simulink library "vmc"  (R2021b)
settings: Solver=VariableStepAuto  StartTime=0.0  StopTime=10.0  RelTol=1e-3
undefined symbols (not defined in the file or in its folder): AVMC_ACCDeltaTqIGain4OVRD_X_kph, AVMC_ACCDeltaTqIGain4OVRD_Y_mps2, AVMC_ACCDeltaTqIGain_X_kph, AVMC_ACCDeltaTqIGain_Y_mps2, AVMC_ACCDeltaTqPGain_X_kph, AVMC_ACCDeltaTqPGain_Y_kph, AVMC_ACCLongSteadyCtrl_X_kph, AVMC_ADSPosGFBDeltaTq_X_kph, AVMC_ADSPosGFBDeltaTq_Y_mps2, AVMC_AggressJerkPCT4AT_X_kph, AVMC_AggressJerkPCT_X_kph, AVMC_AggressLimitPCT4AT_X_kph, AVMC_AggressLimitPCT_X_kph, AVMC_CCLongSteadyCtrl_X_kph, AVMC_DISCDeltaTqIGain_X_kph, AVMC_DISCDeltaTqIGain_Y_mps2, AVMC_DISCDeltaTqPGain_X_kph, AVMC_DISCDeltaTqPGain_Y_kph, AVMC_ESCRegenOut_X_kph, AVMC_ESCRegenOut_Y_Deg, AVMC_ESCRegenOutEnSpd_X_Deg, AVMC_ISOAccLimit_X_mps, AVMC_ISODecLimit_X_mps, AVMC_ISOJerk_X_mps, AVMC_LatESCRegenOut_X_kph, AVMC_LatESCRegenOut_Y_Deg, AVMC_LongAccDeadZone_X_kph, AVMC_LongAccFiltTsforP2_X_Gps, AVMC_MCPresBaseTq_X_bar, AVMC_MSALongSteadyCtrl_X_kph, AVMC_MSAPedalOvrd_X_kph, AVMC_MSASpdBand_X_kph, AVMC_MSATqDownEndTq_X_kph, AVMC_MSATqDownTime_X_kph, AVMC_OPDDisSlideRate_X_Deg, AVMC_OVRD2ActSR2FCMCMD_X_mps2, AVMC_PedalTqRWhlRatio_X_Nm, AVMC_PedalTqRWhlRatio_Y_gps, AVMC_PedalTqRWhlSlipGain_X_rat, AVMC_PedalTqRWhlSlipGain_Y_kph, AVMC_PedalTqRWhSTRGGain_X_deg, AVMC_PedalTqRWhSTRGGain_Y_kph, AVMC_RDCDetectTime_X_kph, AVMC_RDCDetectTime_Y_pct, AVMC_RDCEnSlideRate_X_Deg, AVMC_RearWhlTqRatio_X_Nm, AVMC_RearWhlTqRatio_Y_gps, AVMC_RearWhlTqSlipGain_X_rat, AVMC_RearWhlTqSlipGain_Y_kph, AVMC_RearWhlTqSTRGGain_X_deg, AVMC_RearWhlTqSTRGGain_Y_kph, AVMC_ReqBrkJoinDecSR_X_mps2, AVMC_SoftJerkPCT_X_kph, AVMC_SoftLimitPCT_X_kph, AVMC_StESCYaw_X_kph, AVMC_StESCYaw_Y_Deg, AVMC_StESCYawCom_X_kph, AVMC_StESCYawCom_Y_Gps, AVMC_TMSpdBaseTq_X_rpm, AVMC_VehHoldDecCtrlTime2_X_kph ... (+411)
libraries: hcu_lib x108, simulink x82, tqr x1, simulink_extras x1
(part 3 of 14)

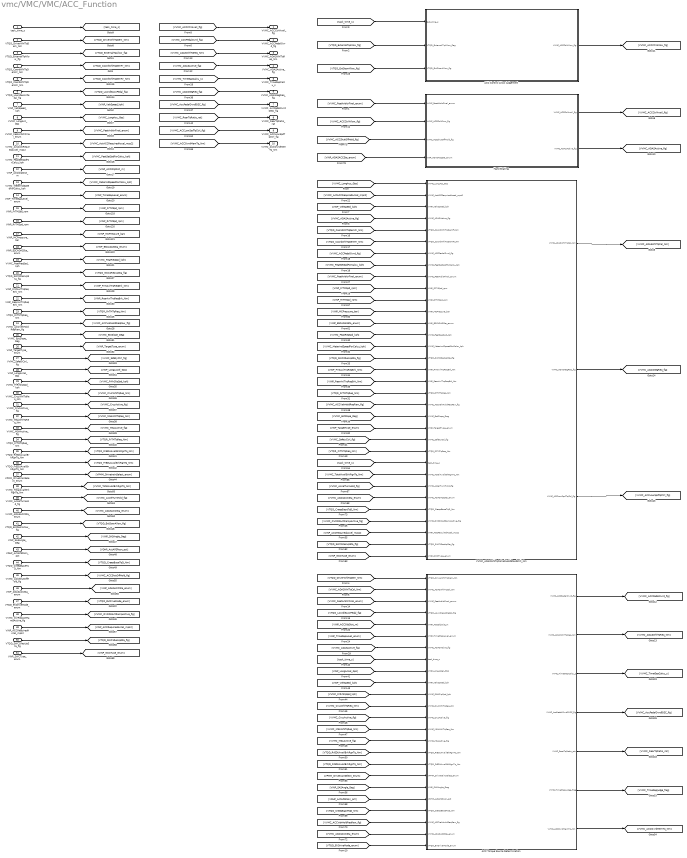
== system vmc/VMC/VMC/ACC_Function ==
  task_time_s : Inport
  VTQD_DriverWhlTqDem_Nm : Inport  Port=2
  VTQD_ExternalTqAllow_flg : Inport  Port=3
  VTQD_CoordWhlTqDemFr_Nm : Inport  Port=4
  VTQD_CoordWhlTqDemRr_Nm : Inport  Port=5
  VTQD_LowIdleAccPedal_flg : Inport  Port=6
  VINP_VehSpeed_kph : Inport  Port=7
  VVMC_LongAcc_Gps : Inport  Port=8
  VVMC_FeatArbitrFinal_enum : Inport  Port=9
  VVMC_ActACCRequiredAccel_mps2 : Inport  Port=10
  VVMC_FeatSetSpdForCalcu_kph : Inport  Port=11
  VINP_ACCObjDist_m : Inport  Port=12
  VVMC_MeterIndSpeedForCalcu_kph : Inport  Port=13
  VINP_TimeGapLevel_enum : Inport  Port=14
  VINP_FrTMSpd_rpm : Inport  Port=15
  VINP_RrTMSpd_rpm : Inport  Port=16
  VINP_MCPressure_bar : Inport  Port=17
  VINP_ESCADASSta_enum : Inport  Port=18
  VVMC_FeatReqSpd_kph : Inport  Port=19
  VTQD_SWC2ResUpSta_flg : Inport  Port=20
  VINP_FrntAxlTrqReqBrk_Nm : Inport  Port=21
  VINP_RearAxlTrqReqBrk_Nm : Inport  Port=22
  VTQR_RrTMTqReq_Nm : Inport  Port=23
  VVMC_ACCVehHoldReqRaw_flg : Inport  Port=24
  VVMC_EstSlope_Deg : Inport  Port=25
  VINP_TargetType_enum : Inport  Port=26
  VVMC_SafetyCtrl_flg : Inport  Port=27
  VINP_LongAccel_Gps : Inport  Port=28
  VVMC_FrRrSlipSpd_kph : Inport  Port=29
  VVMC_CruzWhlTqReq_Nm : Inport  Port=30
  VVMC_CruzActive_flg : Inport  Port=31
  VVMC_MSAWhlTqReq_Nm : Inport  Port=32
  VVMC_MSAActive_flg : Inport  Port=33
  VTQR_FrTMTqReq_Nm : Inport  Port=34
  VTQD_RrEDUAvailBrkRgnTq_Nm : Inport  Port=35
  VTQD_FrEDUAvailBrkRgnTq_Nm : Inport  Port=36
  VPMM_DrivetrainSelect_enum : Inport  Port=37
  VVMC_TotalAvailBrkRgnTq_Nm : Inport  Port=38
  VVMC_AccelTurnHold_flg : Inport  Port=39
  VVMC_ADASACCSta_enum : Inport  Port=40
  VTQD_ExtDoorAllow_flg : Inport  Port=41
  VINP_SASAngle_Deg : Inport  Port=42
  VDHP_ActAPSPosn_pct : Inport  Port=43
  VTQD_CreepBaseTqD_Nm : Inport  Port=44
  VVMC_ACCShutOffHold_flg : Inport  Port=45
  VINP_ADASACCSta_enum : Inport  Port=46
  VTQD_EVDriveMode_enum : Inport  Port=47
  VVMC_OVRD2ActRampActive_flg : Inport  Port=48
  VINP_ACCRequiredAccel_mps2 : Inport  Port=49
  VTQD_SWC1ResUpSta_flg : Inport  Port=50
  VINP_SWCType_enum : Inport  Port=51
  ACC Control Allow Judgement : Subsystem
  ACC Torque Source Determination : Subsystem
  Hand Shaking : Subsystem
  VVMC_ADASWhlTqCalVehHoldStandstill_Nm : Subsystem
  VVMC_ACCCtrlAvail_flg : Outport
  VVMC_ACCPedalOvrd_flg : Outport  Port=2
  VVMC_ADASWhlTqReq_Nm : Outport  Port=3
  VVMC_ADASActive_flg : Outport  Port=4
  VVMC_TimeGapCalcu_s : Outport  Port=5
  VVMC_ADASNegReq_flg : Outport  Port=6
  VVMC_AccPedalOvrdDISC_flg : Outport  Port=7
  VVMC_RearTqRatio_rat : Outport  Port=8
  VVMC_ACCLowSpdTqCtrl_flg : Outport  Port=9
  VVMC_ACCOvrdMemTq_Nm : Outport  Port=10
  wires:
  [VVMC_FeatReqSpd_kph] -> VVMC_ADASWhlTqCalVehHoldStandstill_Nm/14(VVMC_FeatReqSpd_kph)
  VVMC_FeatReqSpd_kph/1 -> [VVMC_FeatReqSpd_kph]
  [VVMC_ADASActive_flg] -> ACC Torque Source Determination/7(VVMC_ADASActive_flg)
  [VINP_ESCADASSta_enum] -> VVMC_ADASWhlTqCalVehHoldStandstill_Nm/13(VINP_ESCADASSta_enum)
  [VINP_MCPressure_bar] -> VVMC_ADASWhlTqCalVehHoldStandstill_Nm/12(VINP_MCPressure_bar)
  [VINP_RrTMSpd_rpm] -> VVMC_ADASWhlTqCalVehHoldStandstill_Nm/11(VINP_RrTMSpd_rpm)
  [VINP_FrTMSpd_rpm] -> VVMC_ADASWhlTqCalVehHoldStandstill_Nm/10(VINP_FrTMSpd_rpm)
  VINP_FrTMSpd_rpm/1 -> [VINP_FrTMSpd_rpm]
  VINP_RrTMSpd_rpm/1 -> [VINP_RrTMSpd_rpm]
  VINP_MCPressure_bar/1 -> [VINP_MCPressure_bar]
  VINP_ESCADASSta_enum/1 -> [VINP_ESCADASSta_enum]
  [VVMC_FeatArbitrFinal_enum] -> VVMC_ADASWhlTqCalVehHoldStandstill_Nm/9(VVMC_FeatArbitrFinal_enum)
  [VTQD_ExternalTqAllow_flg] -> ACC Control Allow Judgement/2(VTQD_ExternalTqAllow_flag)
  ACC Control Allow Judgement/1(VVMC_ACCCtrlAllow_flg) -> [VVMC_ACCCtrlAllow_flg]
  [task_time_s] -> ACC Control Allow Judgement/1(task_time_s)
  [VVMC_TimeGapCalcu_s] -> VVMC_TimeGapCalcu_s/1
  ACC Torque Source Determination/3(VVMC_TimeGapCalcu_s) -> [VVMC_TimeGapCalcu_s]
  [VINP_TimeGapLevel_enum] -> ACC Torque Source Determination/6(VINP_TimeGapLevel_enum)
  [VINP_ACCObjDist_m] -> ACC Torque Source Determination/5(VINP_ACCObjDist_m)
  VINP_TimeGapLevel_enum/1 -> [VINP_TimeGapLevel_enum]
  VINP_ACCObjDist_m/1 -> [VINP_ACCObjDist_m]
  VVMC_MeterIndSpeedForCalcu_kph/1 -> [VVMC_MeterIndSpeedForCalcu_kph]
  [VVMC_ACCPedalOvrd_flg] -> VVMC_ACCPedalOvrd_flg/1
  Hand Shaking/1(VVMC_ACCCtrlAvail_flg) -> [VVMC_ACCCtrlAvail_flg]
  VVMC_LongAcc_Gps/1 -> [VVMC_LongAcc_Gps]
  VVMC_FeatArbitrFinal_enum/1 -> [VVMC_FeatArbitrFinal_enum]
  VVMC_ActACCRequiredAccel_mps2/1 -> [VVMC_ActACCRequiredAccel_mps2]
  [VVMC_ACCCtrlAvail_flg] -> VVMC_ACCCtrlAvail_flg/1
  VTQD_ExternalTqAllow_flg/1 -> [VTQD_ExternalTqAllow_flg]
  VINP_VehSpeed_kph/1 -> [VINP_VehSpeed_kph]
  VTQD_DriverWhlTqDem_Nm/1 -> [VTQD_DriverWhlTqDem_Nm]
  [VVMC_LongAcc_Gps] -> VVMC_ADASWhlTqCalVehHoldStandstill_Nm/1(VVMC_LongAcc_Gps)
  [VVMC_ActACCRequiredAccel_mps2] -> VVMC_ADASWhlTqCalVehHoldStandstill_Nm/2(VVMC_ActACCRequiredAccel_mps2)
  [VINP_VehSpeed_kph] -> VVMC_ADASWhlTqCalVehHoldStandstill_Nm/3(VINP_VehSpeed_kph)
  VVMC_ADASWhlTqCalVehHoldStandstill_Nm/1(VVMC_ADASWhlTqCal_Nm) -> [VVMC_ADASWhlTqCal_Nm]
  [VTQD_DriverWhlTqDem_Nm] -> ACC Torque Source Determination/1(VTQD_DriverWhlTqDem_Nm)
  [VVMC_ADASWhlTqCal_Nm] -> ACC Torque Source Determination/2(VVMC_ADASWhlTqCal_Nm)
  ACC Torque Source Determination/1(VVMC_ACCPedalOvrd_flg) -> [VVMC_ACCPedalOvrd_flg]
  [VVMC_FeatArbitrFinal_enum] -> Hand Shaking/1(VVMC_FeatArbitrFinal_enum)
  Hand Shaking/2(VVMC_ADASActive_flg) -> [VVMC_ADASActive_flg]
  [VVMC_ADASActive_flg] -> VVMC_ADASWhlTqCalVehHoldStandstill_Nm/4(VVMC_ADASActive_flg)
  task_time_s/1 -> [task_time_s]
  [VVMC_ACCCtrlAllow_flg] -> Hand Shaking/2(VVMC_ACCCtrlAllow_flg)
  [VVMC_ADASActive_flg] -> VVMC_ADASActive_flg/1
  ACC Torque Source Determination/2(VVMC_ADASWhlTqReq_Nm) -> [VVMC_ADASWhlTqReq_Nm]
  [VVMC_ADASWhlTqReq_Nm] -> VVMC_ADASWhlTqReq_Nm/1
  [VTQD_CoordWhlTqDemFr_Nm] -> VVMC_ADASWhlTqCalVehHoldStandstill_Nm/5(VTQD_CoordWhlTqDemFr_Nm)
  [VTQD_CoordWhlTqDemRr_Nm] -> VVMC_ADASWhlTqCalVehHoldStandstill_Nm/6(VTQD_CoordWhlTqDemRr_Nm)
  VTQD_CoordWhlTqDemRr_Nm/1 -> [VTQD_CoordWhlTqDemRr_Nm]
  VTQD_CoordWhlTqDemFr_Nm/1 -> [VTQD_CoordWhlTqDemFr_Nm]
  [VVMC_ACCPedalOvrd_flg] -> VVMC_ADASWhlTqCalVehHoldStandstill_Nm/7(VVMC_ACCPedalOvrd_flg)
  [VVMC_FeatArbitrFinal_enum] -> ACC Torque Source Determination/3(VVMC_FeatArbitrFinal_enum)
  VTQD_LowIdleAccPedal_flg/1 -> [VTQD_LowIdleAccPedal_flg]
  [VTQD_LowIdleAccPedal_flg] -> ACC Torque Source Determination/4(VTQD_LowIdleAccPedal_flg)
  VVMC_FeatSetSpdForCalcu_kph/1 -> [VVMC_FeatSetSpdForCalcu_kph]
  [VVMC_FeatSetSpdForCalcu_kph] -> VVMC_ADASWhlTqCalVehHoldStandstill_Nm/8(VVMC_FeatSetSpdForCalcu_kph)
  VTQD_SWC2ResUpSta_flg/1 -> [VTQD_SWC2ResUpSta_flg]
  VINP_FrntAxlTrqReqBrk_Nm/1 -> [VINP_FrntAxlTrqReqBrk_Nm]
  VINP_RearAxlTrqReqBrk_Nm/1 -> [VINP_RearAxlTrqReqBrk_Nm]
  [VVMC_MeterIndSpeedForCalcu_kph] -> VVMC_ADASWhlTqCalVehHoldStandstill_Nm/15(VVMC_MeterIndSpeedForCalcu_kph)
  [VTQD_SWC2ResUpSta_flg] -> VVMC_ADASWhlTqCalVehHoldStandstill_Nm/16(VTQD_SWC2ResUpSta_flg)
  [VINP_FrntAxlTrqReqBrk_Nm] -> VVMC_ADASWhlTqCalVehHoldStandstill_Nm/17(VINP_FrntAxlTrqReqBrk_Nm)
  [VINP_RearAxlTrqReqBrk_Nm] -> VVMC_ADASWhlTqCalVehHoldStandstill_Nm/18(VINP_RearAxlTrqReqBrk_Nm)
  VVMC_ADASWhlTqCalVehHoldStandstill_Nm/2(VVMC_ADASNegReq_flg) -> [VVMC_ADASNegReq_flg]
  [VVMC_ADASNegReq_flg] -> VVMC_ADASNegReq_flg/1
  VTQR_RrTMTqReq_Nm/1 -> [VTQR_RrTMTqReq_Nm]
  [VTQR_RrTMTqReq_Nm] -> VVMC_ADASWhlTqCalVehHoldStandstill_Nm/19(VTQR_RrTMTqReq_Nm)
  ACC Torque Source Determination/4(VVMC_AccPedalOvrdDISC_flg) -> [VVMC_AccPedalOvrdDISC_flg]
  [VVMC_AccPedalOvrdDISC_flg] -> VVMC_AccPedalOvrdDISC_flg/1
  VVMC_ACCVehHoldReqRaw_flg/1 -> [VVMC_ACCVehHoldReqRaw_flg]
  [VVMC_ACCVehHoldReqRaw_flg] -> VVMC_ADASWhlTqCalVehHoldStandstill_Nm/20(VVMC_ACCVehHoldReqRaw_flg)
  VVMC_EstSlope_Deg/1 -> [VVMC_EstSlope_Deg]
  [VVMC_EstSlope_Deg] -> VVMC_ADASWhlTqCalVehHoldStandstill_Nm/21(VVMC_EstSlope_Deg)
  [VINP_TargetType_enum] -> VVMC_ADASWhlTqCalVehHoldStandstill_Nm/22(VINP_TargetType_enum)
  VINP_TargetType_enum/1 -> [VINP_TargetType_enum]
  [task_time_s] -> ACC Torque Source Determination/8(task_time_s)
  VVMC_SafetyCtrl_flg/1 -> [VVMC_SafetyCtrl_flg]
  [VVMC_SafetyCtrl_flg] -> VVMC_ADASWhlTqCalVehHoldStandstill_Nm/23(VVMC_SafetyCtrl_flg)
  [VINP_LongAccel_Gps] -> ACC Torque Source Determination/9(VINP_LongAccel_Gps)
  ACC Torque Source Determination/5(VVMC_RearTqRatio_rat) -> [VVMC_RearTqRatio_rat]
  [VVMC_RearTqRatio_rat] -> VVMC_RearTqRatio_rat/1
  VINP_LongAccel_Gps/1 -> [VINP_LongAccel_Gps]
  VVMC_FrRrSlipSpd_kph/1 -> [VVMC_FrRrSlipSpd_kph]
  [VINP_VehSpeed_kph] -> ACC Torque Source Determination/10(VINP_VehSpeed_kph)
  [VVMC_FrRrSlipSpd_kph] -> ACC Torque Source Determination/11(VVMC_FrRrSlipSpd_kph)
  VVMC_MSAActive_flg/1 -> [VVMC_MSAActive_flg]
  VVMC_MSAWhlTqReq_Nm/1 -> [VVMC_MSAWhlTqReq_Nm]
  VVMC_CruzActive_flg/1 -> [VVMC_CruzActive_flg]
  VVMC_CruzWhlTqReq_Nm/1 -> [VVMC_CruzWhlTqReq_Nm]
  [VVMC_CruzWhlTqReq_Nm] -> ACC Torque Source Determination/12(VVMC_CruzWhlTqReq_Nm)
  [VVMC_CruzActive_flg] -> ACC Torque Source Determination/13(VVMC_CruzActive_flg)
  [VVMC_MSAWhlTqReq_Nm] -> ACC Torque Source Determination/14(VVMC_MSAWhlTqReq_Nm)
  [VVMC_MSAActive_flg] -> ACC Torque Source Determination/15(VVMC_MSAActive_flg)
  [VTQR_FrTMTqReq_Nm] -> VVMC_ADASWhlTqCalVehHoldStandstill_Nm/24(VTQR_FrTMTqReq_Nm)
  VTQR_FrTMTqReq_Nm/1 -> [VTQR_FrTMTqReq_Nm]
  VTQD_RrEDUAvailBrkRgnTq_Nm/1 -> [VTQD_RrEDUAvailBrkRgnTq_Nm]
  VTQD_FrEDUAvailBrkRgnTq_Nm/1 -> [VTQD_FrEDUAvailBrkRgnTq_Nm]
  [VTQD_RrEDUAvailBrkRgnTq_Nm] -> ACC Torque Source Determination/16(VTQD_RrEDUAvailBrkRgnTq_Nm)
  [VTQD_FrEDUAvailBrkRgnTq_Nm] -> ACC Torque Source Determination/17(VTQD_FrEDUAvailBrkRgnTq_Nm)
  VVMC_ADASWhlTqCalVehHoldStandstill_Nm/3(VVMC_ACCLowSpdTqCtrl_flg) -> [VVMC_ACCLowSpdTqCtrl_flg]
  [VVMC_ACCLowSpdTqCtrl_flg] -> VVMC_ACCLowSpdTqCtrl_flg/1
  VPMM_DrivetrainSelect_enum/1 -> [VPMM_DrivetrainSelect_enum]
  [VPMM_DrivetrainSelect_enum] -> ACC Torque Source Determination/18(VPMM_DrivetrainSelect_enum)
  [task_time_s] -> VVMC_ADASWhlTqCalVehHoldStandstill_Nm/25(task_time_s)
  VVMC_TotalAvailBrkRgnTq_Nm/1 -> [VVMC_TotalAvailBrkRgnTq_Nm]
  [VVMC_TotalAvailBrkRgnTq_Nm] -> VVMC_ADASWhlTqCalVehHoldStandstill_Nm/26(VVMC_TotalAvailBrkRgnTq_Nm)
  VVMC_AccelTurnHold_flg/1 -> [VVMC_AccelTurnHold_flg]
  [VVMC_AccelTurnHold_flg] -> VVMC_ADASWhlTqCalVehHoldStandstill_Nm/27(VVMC_AccelTurnHold_flg)
  VVMC_ADASACCSta_enum/1 -> [VVMC_ADASACCSta_enum]
  [VVMC_ADASACCSta_enum] -> VVMC_ADASWhlTqCalVehHoldStandstill_Nm/28(VVMC_ADASACCSta_enum)
  ACC Torque Source Determination/6(VVMC_TimeGapJudge_flag) -> [VVMC_TimeGapJudge_flag]
  [VTQD_ExtDoorAllow_flg] -> ACC Control Allow Judgement/3(VTQD_ExtDoorAllow_flg)
  VTQD_ExtDoorAllow_flg/1 -> [VTQD_ExtDoorAllow_flg]
  [VINP_SASAngle_Deg] -> ACC Torque Source Determination/19(VINP_SASAngle_Deg)
  VINP_SASAngle_Deg/1 -> [VINP_SASAngle_Deg]
  [VDHP_ActAPSPosn_pct] -> ACC Torque Source Determination/20(VDHP_ActAPSPosn_pct)
  VDHP_ActAPSPosn_pct/1 -> [VDHP_ActAPSPosn_pct]
  VTQD_CreepBaseTqD_Nm/1 -> [VTQD_CreepBaseTqD_Nm]
  [VTQD_CreepBaseTqD_Nm] -> ACC Torque Source Determination/21(VTQD_CreepBaseTqD_Nm)
  [VVMC_ACCOvrdMemTq_Nm] -> VVMC_ACCOvrdMemTq_Nm/1
  ACC Torque Source Determination/7(VVMC_ACCOvrdMemTq_Nm) -> [VVMC_ACCOvrdMemTq_Nm]
  [VVMC_ACCVehHoldReqRaw_flg] -> ACC Torque Source Determination/22(VVMC_ACCVehHoldReqRaw_flg)
  [VVMC_ADASACCSta_enum] -> ACC Torque Source Determination/23(VVMC_ADASACCSta_enum)
  [VTQD_CreepBaseTqD_Nm] -> VVMC_ADASWhlTqCalVehHoldStandstill_Nm/29(VTQD_CreepBaseTqD_Nm)
  VVMC_ACCShutOffHold_flg/1 -> [VVMC_ACCShutOffHold_flg]
  [VVMC_ACCShutOffHold_flg] -> Hand Shaking/3(VVMC_ACCShutOffHold_flg)
  VINP_ADASACCSta_enum/1 -> [VINP_ADASACCSta_enum]
  [VINP_ADASACCSta_enum] -> Hand Shaking/4(VINP_ADASACCSta_enum)
  VTQD_EVDriveMode_enum/1 -> [VTQD_EVDriveMode_enum]
  [VTQD_EVDriveMode_enum] -> ACC Torque Source Determination/24(VTQD_EVDriveMode_enum)
  VVMC_OVRD2ActRampActive_flg/1 -> [VVMC_OVRD2ActRampActive_flg]
  [VVMC_OVRD2ActRampActive_flg] -> VVMC_ADASWhlTqCalVehHoldStandstill_Nm/30(VVMC_OVRD2ActRampActive_flg)
  VINP_ACCRequiredAccel_mps2/1 -> [VINP_ACCRequiredAccel_mps2]
  [VINP_ACCRequiredAccel_mps2] -> VVMC_ADASWhlTqCalVehHoldStandstill_Nm/31(VINP_ACCRequiredAccel_mps2)
  VTQD_SWC1ResUpSta_flg/1 -> [VTQD_SWC1ResUpSta_flg]
  [VTQD_SWC1ResUpSta_flg] -> VVMC_ADASWhlTqCalVehHoldStandstill_Nm/32(VTQD_SWC1ResUpSta_flg)
  VINP_SWCType_enum/1 -> [VINP_SWCType_enum]
  [VINP_SWCType_enum] -> VVMC_ADASWhlTqCalVehHoldStandstill_Nm/33(VINP_SWCType_enum)

== system vmc/VMC/VMC/APS function ==
  VTQD_ExternalTqAllow_flg : Inport
  VTQD_ExtShiftAllow_flg : Inport  Port=2
  VTQD_ExtDoorAllow_flg : Inport  Port=3
  VTQD_GearActualPosn_enum : Inport  Port=4
  VINP_APSVMCReqA_flg : Inport  Port=5
  VINP_APSShiftPosnReq_enum : Inport  Port=6
  VINP_APSSpeedCMD_kph : Inport  Port=7
  task_time_s : Inport  Port=8
  VINP_SCPSystemMode_enum : Inport  Port=9
  VVMC_ADASActive_flg : Inport  Port=10
  VTQD_APSStaSys_enum : Inport  Port=11
  VTQD_APSDecReqA_flg : Inport  Port=12
  VTQD_APSDecReq_mps2 : Inport  Port=13
  VTQD_APSReq_enum : Inport  Port=14
  VINP_APSStaSystem_enum : Inport  Port=15
  VINP_APSDecReqA_flg : Inport  Port=16
  VINP_APSDecReq_mps2 : Inport  Port=17
  VINP_APSReq_enum : Inport  Port=18
  VINP_VehSpeed_kph : Inport  Port=19
  VVMC_CruzActive_flg : Inport  Port=20
  VINP_CAASVMCReqA_flg : Inport  Port=21
  VINP_ADASACCSta_enum : Inport  Port=22
  VINP_BrkSwSta_flg : Inport  Port=23
  VINP_MCPressure_bar : Inport  Port=24
  VINP_BrkPedalPos_pct : Inport  Port=25
  VINP_ACCObjDist_m : Inport  Port=26
  VVMC_MeterIndSpeedForCalcu_kph : Inport  Port=27
  VDDM_VCURAPSErrLv2_flg : Inport  Port=28
  VDDM_VCURAPSErrLv3_flg : Inport  Port=29
  VTQD_EPBCarWashMode_flg : Inport  Port=30
  CAAS HandShake : Subsystem
  Command Determination1 : Subsystem
  Hand Shake : Subsystem
  Signal Rounting1 : Subsystem
  Subsystem : Subsystem
  VVMC_APSCtrlAvail_flg : Outport
  VVMC_APSActive_flg : Outport  Port=2
  VVMC_CAASCtrlAvail_flg : Outport  Port=3
  VVMC_CAASActive_flg : Outport  Port=4
  VVMC_APSSpeedCMD_kph : Outport  Port=5
  VVMC_APSShiftPosnReq_enum : Outport  Port=6
  VVMC_APSStaSys_enum : Outport  Port=7
  VVMC_APSDecReqA_flg : Outport  Port=8
  VVMC_APSDecReq_mps2 : Outport  Port=9
  VVMC_APSReq_enum : Outport  Port=10
  VVMC_SetACCDisableAPS_flg : Outport  Port=11
  wires:
  task_time_s/1 -> [task_time_s]
  VINP_APSSpeedCMD_kph/1 -> [VINP_APSSpeedCMD_kph]
  VINP_APSShiftPosnReq_enum/1 -> [VINP_APSShiftPosnReq_enum]
  VINP_APSVMCReqA_flg/1 -> [VINP_APSVMCReqA_flg]
  VVMC_ADASActive_flg/1 -> [VVMC_ADASActive_flg]
  VTQD_ExtDoorAllow_flg/1 -> [VTQD_ExtDoorAllow_flg]
  VTQD_ExternalTqAllow_flg/1 -> [VTQD_ExternalTqAllow_flg]
  VTQD_ExtShiftAllow_flg/1 -> [VTQD_ExtShiftAllow_flg]
  VTQD_GearActualPosn_enum/1 -> [VTQD_GearActualPosn_enum]
  VINP_SCPSystemMode_enum/1 -> [VINP_SCPSystemMode_enum]
  VTQD_APSStaSys_enum/1 -> [VTQD_APSStaSys_enum]
  VTQD_APSDecReq_mps2/1 -> [VTQD_APSDecReq_mps2]
  VTQD_APSDecReqA_flg/1 -> [VTQD_APSDecReqA_flg]
  VTQD_APSReq_enum/1 -> [VTQD_APSReq_enum]
  Hand Shake/1(VVMC_APSCtrlAvail_flg) -> VVMC_APSCtrlAvail_flg/1
  [VTQD_ExtDoorAllow_flg] -> Hand Shake/6(VTQD_ExtDoorAllow_flg)
  Hand Shake/2(VVMC_APSActive_flg) -> VVMC_APSActive_flg/1, [VVMC_APSActive_flg]
  [VVMC_CruzActive_flg] -> CAAS HandShake/3(VVMC_CruzActive_flg)
  [VINP_VehSpeed_kph] -> CAAS HandShake/1(VINP_VehSpeed_kph)
  [VVMC_ADASActive_flg] -> CAAS HandShake/2(VVMC_ADASActive_flg)
  [VINP_APSVMCReqA_flg] -> Hand Shake/4(VINP_APSVMCReqA_flg)
  CAAS HandShake/1(VVMC_CAASCtrlAvail_flg) -> VVMC_CAASCtrlAvail_flg/1
  [task_time_s] -> CAAS HandShake/4(task_time_s)
  [VINP_CAASVMCReqA_flg] -> CAAS HandShake/5(VINP_CAASVMCReqA_flg)
  CAAS HandShake/2(VVMC_CAASActive_flg) -> VVMC_CAASActive_flg/1, [VVMC_CAASActive_flg]
  [VINP_APSStaSystem_enum] -> Hand Shake/5(VINP_APSStaSys_enum)
  [VTQD_ExtShiftAllow_flg] -> Hand Shake/3(VTQD_ExtShiftAllow_flg)
  [task_time_s] -> Hand Shake/1(task_time_s)
  [VTQD_ExternalTqAllow_flg] -> Hand Shake/2(VTQD_ExternalTqAllow_flg)
  Command Determination1/1(VVMC_APSSpeedCMD_kph) -> VVMC_APSSpeedCMD_kph/1
  [VVMC_CAASActive_flg] -> Signal Rounting1/5(VVMC_CAASActive_flg)
  [VVMC_APSActive_flg] -> Command Determination1/1(VVMC_APSActive_flg)
  Signal Rounting1/2(VVMC_APSDecReqA_flg) -> VVMC_APSDecReqA_flg/1
  Signal Rounting1/3(VVMC_APSDecReq_mps2) -> VVMC_APSDecReq_mps2/1
  [VVMC_ADASActive_flg] -> Signal Rounting1/3(VVMC_ADASActive_flg)
  Signal Rounting1/1(VVMC_APSStaSys_enum) -> VVMC_APSStaSys_enum/1
  [VVMC_APSActive_flg] -> Signal Rounting1/2(VVMC_APSActive_flg)
  [VINP_SCPSystemMode_enum] -> Signal Rounting1/1(VINP_SCPSystemMode_enum)
  [VTQD_GearActualPosn_enum] -> Signal Rounting1/4(VTQD_GearActualPosn_enum)
  [VINP_APSStaSystem_enum] -> Command Determination1/2(VINP_APSStaSys_enum)
  [VINP_APSShiftPosnReq_enum] -> Command Determination1/3(VINP_APSShiftPosnReq_enum)
  Command Determination1/2(VVMC_APSShiftPosnReq_enum) -> VVMC_APSShiftPosnReq_enum/1
  [VINP_APSSpeedCMD_kph] -> Command Determination1/4(VINP_APSSpeedCMD_kph)
  Signal Rounting1/4(VVMC_APSReq_enum) -> VVMC_APSReq_enum/1
  VINP_APSDecReq_mps2/1 -> [VINP_APSDecReq_mps2]
  VINP_APSReq_enum/1 -> [VINP_APSReq_enum]
  VINP_APSStaSystem_enum/1 -> [VINP_APSStaSystem_enum]
  VINP_APSDecReqA_flg/1 -> [VINP_APSDecReqA_flg]
  [VTQD_APSStaSys_enum] -> Signal Rounting1/6(VTQD_APSStaSys_enum)
  [VINP_APSStaSystem_enum] -> Signal Rounting1/10(VINP_APSStaSystem_enum)
  [VTQD_APSDecReqA_flg] -> Signal Rounting1/7(VTQD_APSDecReqA_flg)
  [VTQD_APSDecReq_mps2] -> Signal Rounting1/8(VTQD_APSDecReq_mps2)
  [VINP_APSDecReqA_flg] -> Signal Rounting1/11(VINP_APSDecReqA_flg)
  [VINP_APSDecReq_mps2] -> Signal Rounting1/12(VINP_APSDecReq_mps2)
  [VINP_APSReq_enum] -> Signal Rounting1/13(VINP_APSReq_enum)
  [VTQD_APSReq_enum] -> Signal Rounting1/9(VTQD_APSReq_enum)
  VINP_VehSpeed_kph/1 -> [VINP_VehSpeed_kph]
  VVMC_CruzActive_flg/1 -> [VVMC_CruzActive_flg]
  VINP_CAASVMCReqA_flg/1 -> [VINP_CAASVMCReqA_flg]
  [VTQD_APSDecReqA_flg] -> Subsystem/5(VTQD_APSDecReqA_flg)
  [VINP_BrkPedalPos_pct] -> Subsystem/4(VINP_BrkPedalPos_pct)
  [VINP_MCPressure_bar] -> Subsystem/2(VINP_MCPressure_bar)
  [VINP_BrkSwSta_flg] -> Subsystem/3(VINP_BrkSwSta_flg)
  [VINP_ACCObjDist_m] -> Subsystem/6(VINP_ACCObjDist_m)
  [VVMC_MeterIndSpeedForCalcu_kph] -> Subsystem/7(VVMC_MeterIndSpeedForCalcu_kph)
  [VINP_ADASACCSta_enum] -> Subsystem/1(VINP_ADASACCSta_enum)
  Subsystem/1(VVMC_SetACCDisableAPS_flg) -> VVMC_SetACCDisableAPS_flg/1, [VVMC_SetACCDisableAPS_flg]
  VINP_ADASACCSta_enum/1 -> [VINP_ADASACCSta_enum]
  VINP_BrkSwSta_flg/1 -> [VINP_BrkSwSta_flg]
  VINP_MCPressure_bar/1 -> [VINP_MCPressure_bar]
  VINP_BrkPedalPos_pct/1 -> [VINP_BrkPedalPos_pct]
  VINP_ACCObjDist_m/1 -> [VINP_ACCObjDist_m]
  VVMC_MeterIndSpeedForCalcu_kph/1 -> [VVMC_MeterIndSpeedForCalcu_kph]
  [VVMC_SetACCDisableAPS_flg] -> Signal Rounting1/14(VVMC_SetACCDisableAPS_flg)
  [VINP_VehSpeed_kph] -> Subsystem/8(VINP_VehSpeed_kph)
  [VDDM_VCURAPSErrLv3_flg] -> Hand Shake/9(VDDM_VCURAPSErrLv3_flg)
  [VDDM_VCURAPSErrLv2_flg] -> Hand Shake/8(VDDM_VCURAPSErrLv2_flg)
  [VTQD_GearActualPosn_enum] -> Hand Shake/7(VTQD_GearActualPosn_enum)
  [VTQD_EPBCarWashMode_flg] -> Hand Shake/10(VTQD_EPBCarWashMode_flg)
  VDDM_VCURAPSErrLv3_flg/1 -> [VDDM_VCURAPSErrLv3_flg]
  VTQD_EPBCarWashMode_flg/1 -> [VTQD_EPBCarWashMode_flg]
  VDDM_VCURAPSErrLv2_flg/1 -> [VDDM_VCURAPSErrLv2_flg]

== system vmc/VMC/VMC/CruiseControlFunction ==
  VTQD_ExternalTqAllow_flg : Inport
  VTQD_DriverWhlTqDem_Nm : Inport  Port=2
  VTQD_LowIdleAccPedal_flg : Inport  Port=3
  <VTQD_SpdCtrlMode_enum> : Inport  Port=4
  VTQD_SWC1ResUpSta_flg : Inport  Port=5
  VTQD_SWC1SetdownSta_flg : Inport  Port=6
  VTQD_SWC1CANCELSta_flg : Inport  Port=7
  VINP_BrakeSWGPIO_flg : Inport  Port=8
  VINP_BrkSwSta_flg : Inport  Port=9
  VINP_VehSpeed_kph : Inport  Port=10
  VVMC_LongAcc_Gps : Inport  Port=11
  VVMC_FeatSetSpdForCalcu_kph : Inport  Port=12
  VVMC_FeatArbitrFinal_enum : Inport  Port=13
  VINP_ADASAEBSta_enum : Inport  Port=14
  VTQD_GearActualPosn_enum : Inport  Port=15
  VVMC_SafetyCtrl_flg : Inport  Port=16
  VTQR_FrTMTqReq_Nm : Inport  Port=17
  VTQR_RrTMTqReq_Nm : Inport  Port=18
  VTQD_RegenMode_enum : Inport  Port=19
  VVMC_ActACCRequiredAccel_mps2 : Inport  Port=20
  task_time_s : Inport  Port=21
  VVMC_TotalAvailBrkRgnTq_Nm : Inport  Port=22
  VINP_Distanceunit_flg : Inport  Port=23
  VTQD_ExtDoorAllow_flg : Inport  Port=24
  VVMC_VMCCCCtrlAvail_flg : Inport  Port=25
  VVMC_FeatSetSpdFinal_raw32 : Inport  Port=26
  CCActiveDetermination : Subsystem
  CCDemandTorqueCalculation : Subsystem
  CCTorqueSourceDetermination : Subsystem
  Data Type Conversion : DataTypeConversion  OutDataTypeStr=single
  VVMC_CCCtrlSta_enum : Outport
  VVMC_CCSpdWar_flg : Outport  Port=2
  VVMC_CruzWhlTqReq_Nm : Outport  Port=3
  VVMC_CruzActive_flg : Outport  Port=4
  VVMC_CCPedalOvrd_flg : Outport  Port=5
  wires:
  [VVMC_CCPedalOvrd_flg] -> VVMC_CCPedalOvrd_flg/1
  [VVMC_CCPedalOvrd_flg] -> CCActiveDetermination/12(VVMC_CCPedalOvrd_flg)
  [VINP_ADASAEBSta_enum] -> CCActiveDetermination/11(VINP_ADASAEBSta_enum)
  VINP_ADASAEBSta_enum/1 -> [VINP_ADASAEBSta_enum]
  [VTQD_SpdCtrlMode_enum] -> CCActiveDetermination/1(VTQD_SpdCtrlMode_enum)
  <VTQD_SpdCtrlMode_enum>/1 -> [VTQD_SpdCtrlMode_enum]
  [VVMC_FeatArbitrFinal_enum] -> CCActiveDetermination/2(VVMC_FeatArbitrFinal_enum)
  [VTQD_ExternalTqAllow_flg] -> CCActiveDetermination/3(VTQD_ExternalTqAllow_flg)
  [VTQD_SWC1SetdownSta_flg] -> CCActiveDetermination/4(VTQD_SWC1SetdownSta_flg)
  [VTQD_SWC1ResUpSta_flg] -> CCActiveDetermination/5(VTQD_SWC1ResUpSta_flg)
  [VVMC_FeatSetSpdFinal_raw32] -> CCActiveDetermination/7(VVMC_FeatSetSpdFinal_raw32)
  [VINP_BrakeSWGPIO_flg] -> CCActiveDetermination/8(VINP_BrakeSWGPIO_flg)
  [VTQD_SWC1CANCELSta_flg] -> CCActiveDetermination/9(VTQD_SWC1CANCELSta_flg)
  [VINP_BrkSwSta_flg] -> CCActiveDetermination/10(VINP_BrkSwSta_flg)
  [VVMC_FeatSetSpdForCalcu_kph] -> CCDemandTorqueCalculation/1(VVMC_FeatSetSpdForCalcu_kph)
  [VINP_VehSpeed_kph] -> CCDemandTorqueCalculation/2(VINP_VehSpeed_kph)
  [VVMC_CruzActive_flg] -> CCDemandTorqueCalculation/3(VVMC_CruzActive_flg)
  [VTQD_DriverWhlTqDem_Nm] -> CCTorqueSourceDetermination/1(VTQD_DriverWhlTqDem_Nm)
  [VVMC_CruzWhlTqCal_Nm] -> CCTorqueSourceDetermination/2(VVMC_CruzWhlTqCal_Nm)
  CCActiveDetermination/1(VVMC_CCCtrlSta_enum) -> [VVMC_CCCtrlSta_enum]
  CCActiveDetermination/2(VVMC_CCSpdWar_flg) -> [VVMC_CCSpdWar_flg]
  CCActiveDetermination/3(VVMC_CruzActive_flg) -> [VVMC_CruzActive_flg]
  CCDemandTorqueCalculation/1(VVMC_CruzWhlTqCal_Nm) -> [VVMC_CruzWhlTqCal_Nm]
  CCTorqueSourceDetermination/1(VVMC_CruzWhlTqReq_Nm) -> [VVMC_CruzWhlTqReq_Nm]  "VVMC_CruzWhlTqReq_Nm"
  VTQD_ExternalTqAllow_flg/1 -> [VTQD_ExternalTqAllow_flg]
  VTQD_DriverWhlTqDem_Nm/1 -> [VTQD_DriverWhlTqDem_Nm]
  VTQD_SWC1ResUpSta_flg/1 -> [VTQD_SWC1ResUpSta_flg]
  VTQD_SWC1SetdownSta_flg/1 -> [VTQD_SWC1SetdownSta_flg]
  VTQD_SWC1CANCELSta_flg/1 -> [VTQD_SWC1CANCELSta_flg]
  VINP_BrakeSWGPIO_flg/1 -> [VINP_BrakeSWGPIO_flg]
  VVMC_FeatSetSpdForCalcu_kph/1 -> Data Type Conversion/1
  VINP_BrkSwSta_flg/1 -> [VINP_BrkSwSta_flg]
  VVMC_FeatArbitrFinal_enum/1 -> [VVMC_FeatArbitrFinal_enum]
  VINP_VehSpeed_kph/1 -> [VINP_VehSpeed_kph]
  [VVMC_CCCtrlSta_enum] -> VVMC_CCCtrlSta_enum/1
  [VVMC_CCSpdWar_flg] -> VVMC_CCSpdWar_flg/1
  [VVMC_CruzWhlTqReq_Nm] -> VVMC_CruzWhlTqReq_Nm/1
  Data Type Conversion/1 -> [VVMC_FeatSetSpdForCalcu_kph]  "VVMC_FeatSetSpdForCalcu_kph"
  [VVMC_CruzActive_flg] -> VVMC_CruzActive_flg/1
  VVMC_LongAcc_Gps/1 -> [VVMC_LongAcc_Gps]
  [VVMC_LongAcc_Gps] -> CCDemandTorqueCalculation/4(VVMC_LongAcc_Gps)
  [VINP_VehSpeed_kph] -> CCActiveDetermination/6(VINP_VehSpeed_kph)
  VTQD_LowIdleAccPedal_flg/1 -> [VTQD_LowIdleAccPedal_flg]
  [VTQD_LowIdleAccPedal_flg] -> CCTorqueSourceDetermination/3(VTQD_LowIdleAccPedal_flg)
  CCTorqueSourceDetermination/2(VVMC_CCPedalOvrd_flg) -> [VVMC_CCPedalOvrd_flg]  "VVMC_CCPedalOvrd_flg"
  [VVMC_CCPedalOvrd_flg] -> CCDemandTorqueCalculation/5(VVMC_CCPedalOvrd_flg)
  VTQD_GearActualPosn_enum/1 -> [VTQD_GearActualPosn_enum]
  [VTQD_GearActualPosn_enum] -> CCActiveDetermination/13(VTQD_GearActualPosn_enum)
  [VVMC_SafetyCtrl_flg] -> CCDemandTorqueCalculation/7(VVMC_SafetyCtrl_flg)
  VVMC_SafetyCtrl_flg/1 -> [VVMC_SafetyCtrl_flg]
  [VTQR_FrTMTqReq_Nm] -> CCDemandTorqueCalculation/8(VTQR_FrTMTqReq_Nm)
  [VTQR_RrTMTqReq_Nm] -> CCDemandTorqueCalculation/9(VTQR_RrTMTqReq_Nm)
  VTQR_FrTMTqReq_Nm/1 -> [VTQR_FrTMTqReq_Nm]
  VTQR_RrTMTqReq_Nm/1 -> [VTQR_RrTMTqReq_Nm]
  [VTQD_RegenMode_enum] -> CCTorqueSourceDetermination/4(VTQD_RegenMode_enum)
  [VVMC_FeatArbitrFinal_enum] -> CCTorqueSourceDetermination/5(VVMC_FeatArbitrFinal_enum)
  VTQD_RegenMode_enum/1 -> [VTQD_RegenMode_enum]
  [task_time_s] -> CCTorqueSourceDetermination/6(task_time_s)
  VVMC_ActACCRequiredAccel_mps2/1 -> [VVMC_ActACCRequiredAccel_mps2]
  task_time_s/1 -> [task_time_s]
  [VVMC_ActACCRequiredAccel_mps2] -> CCDemandTorqueCalculation/6(VVMC_ActACCRequiredAccel_mps2)
  VVMC_TotalAvailBrkRgnTq_Nm/1 -> [VVMC_TotalAvailBrkRgnTq_Nm]
  [VVMC_TotalAvailBrkRgnTq_Nm] -> CCDemandTorqueCalculation/10(VVMC_TotalAvailBrkRgnTq_Nm)
  [VINP_Distanceunit_flg] -> CCActiveDetermination/14(VINP_Distanceunit_flg)
  VINP_Distanceunit_flg/1 -> [VINP_Distanceunit_flg]
  VTQD_ExtDoorAllow_flg/1 -> [VTQD_ExtDoorAllow_flg]
  [VTQD_ExtDoorAllow_flg] -> CCActiveDetermination/15(VTQD_ExtDoorAllow_flg)
  VVMC_VMCCCCtrlAvail_flg/1 -> [VVMC_VMCCCCtrlAvail_flg]
  [VVMC_VMCCCCtrlAvail_flg] -> CCActiveDetermination/16(VVMC_VMCCCCtrlAvail_flg)
  VVMC_FeatSetSpdFinal_raw32/1 -> [VVMC_FeatSetSpdFinal_raw32]

== system vmc/VMC/VMC/FeatureSetSpeed ==
  APP_SpdLimit_flg : Inport
  VTQD_SpdCtrlSta_flg : Inport  Port=2
  APP_SpdLimit : Inport  Port=3
  VTQD_SetSpd_kph : Inport  Port=4
  VINP_Distanceunit_flg : Inport  Port=5
  AND : Logic  AllPortsSameDT=off  OutDataTypeStr=boolean
  Cast To Single : DataTypeConversion  OutDataTypeStr=single
  Cast To Single1 : DataTypeConversion  OutDataTypeStr=single
  Constant : Constant  Value=ENUM_SCPCRLSTA_ON
  Constant1 : Constant  Value=ENUM_APPSPDLIMIT_ON
  Constant2 : Constant  Value=ZERO_FLOAT
  Constant3 : Constant  Value=ONE_FLOAT
  Constant4 : Constant  Value=MPH2KPH
  Constant5 : Constant  Value=KVMC_APPSpdLimit_flg_ovrdflg
  Constant6 : Constant  Value=KVMC_APPSpdLimit_flg_ovrdval
  Constant7 : Constant  Value=KVMC_APPSpdLimit_ovrdflg
  Constant8 : Constant  Value=KVMC_APPSpdLimit_ovrdval
  Divide1 : Product  Inputs=**
  Relational Operator : RelationalOperator  Operator=>  OutDataTypeStr=boolean  RndMeth=Simplest
  Round1 : Rounding  Operator=ceil
  SpeedDetermination : Stateflow chart  TreatAsAtomicUnit=on
  Switch : Switch  Criteria=u2 ~= 0
  Switch1 : Switch  Criteria=u2 ~= 0
  u2 > 0 (2) : Switch  Criteria=u2 > Threshold
  VVMC_FeatSetSpdFinal_raw32 : Outport
  VVMC_FeatSetSpdForCalcu_kph : Outport  Port=2
  wires:
  [VTQD_SetSpd_kph] -> SpeedDetermination/4(VTQD_SetSpd_kph)
  Constant2/1 -> SpeedDetermination/7(ZERO_FLOAT)
  Constant6/1 -> Switch/1
  Constant1/1 -> SpeedDetermination/6(ENUM_APPSPDLIMIT_ON)
  Constant5/1 -> Switch/2
  [APP_SpdLimit_flg] -> Switch/3
  SpeedDetermination/1(VVMC_FeatSetSpdFinal_raw32) -> Cast To Single/1
  Constant/1 -> SpeedDetermination/5(ENUM_SCPCRLSTA_ON)
  Switch1/1 -> [VVMC_APPSpdLimit_kph]  "VVMC_APPSpdLimit_kph"
  Constant8/1 -> Switch1/1
  [APP_SpdLimit] -> Switch1/3
  [VTQD_SpdCtrlSta_flg] -> SpeedDetermination/2(VTQD_SpdCtrlSta_flg)
  Constant7/1 -> Switch1/2
  [VVMC_APPSpdLimit_flg] -> SpeedDetermination/1(VVMC_APPSpdLimit_flg)
  Switch/1 -> [VVMC_APPSpdLimit_flg]  "VVMC_APPSpdLimit_flg"
  Cast To Single/1 -> [VVMC_FeatSetSpdFinal_raw32]  "VVMC_FeatSetSpdFinal_raw32"
  [VVMC_APPSpdLimit_kph] -> SpeedDetermination/3(VVMC_APPSpdLimit_kph)
  APP_SpdLimit_flg/1 -> [APP_SpdLimit_flg]
  VTQD_SpdCtrlSta_flg/1 -> [VTQD_SpdCtrlSta_flg]
  APP_SpdLimit/1 -> [APP_SpdLimit]
  VTQD_SetSpd_kph/1 -> [VTQD_SetSpd_kph]
  [VVMC_FeatSetSpdFinal_raw32] -> VVMC_FeatSetSpdFinal_raw32/1
  [VVMC_FeatSetSpdFinal_raw32] -> Divide1/1, u2 > 0 (2)/3
  u2 > 0 (2)/1 -> Cast To Single1/1
  Constant4/1 -> Divide1/2
  Divide1/1 -> u2 > 0 (2)/1
  [VINP_Distanceunit_flg] -> AND/1
  Round1/1 -> [VVMC_FeatSetSpdForCalcu_kph]  "VVMC_FeatSetSpdForCalcu_kph"
  Cast To Single1/1 -> Round1/1
  [VVMC_FeatSetSpdForCalcu_kph] -> VVMC_FeatSetSpdForCalcu_kph/1
  VINP_Distanceunit_flg/1 -> [VINP_Distanceunit_flg]
  Constant3/1 -> Relational Operator/2
  [VVMC_FeatSetSpdFinal_raw32] -> Relational Operator/1
  AND/1 -> u2 > 0 (2)/2
  Relational Operator/1 -> AND/2

== system vmc/VMC/VMC/IMU ==
  VINP_MemOffsetGyroX_raw16 : Inport
  VINP_MemOffsetGyroY_raw16 : Inport  Port=2
  VINP_MemOffsetGyroZ_raw16 : Inport  Port=3
  VINP_MemOffsetAccX_raw16 : Inport  Port=4
  VINP_MemOffsetAccY_raw16 : Inport  Port=5
  VINP_MemOffsetAccZ_raw16 : Inport  Port=6
  VINP_SensingGyroX_raw16 : Inport  Port=7
  VINP_SensingGyroY_raw16 : Inport  Port=8
  VINP_SensingGyroZ_raw16 : Inport  Port=9
  VINP_SensingAccX_raw16 : Inport  Port=10
  VINP_SensingAccY_raw16 : Inport  Port=11
  VINP_SensingAccZ_raw16 : Inport  Port=12
  task_time_s : Inport  Port=13
  Constant : Constant  Value=KVMC_IMUEnaCmd_flg
  IMU memorized offset result : Subsystem
  "IMU sensing result " : Subsystem
  VVMC_IMUEnaCmd_flg : Outport
  VVMC_CalibratedGyroX_Dps : Outport  Port=2
  VVMC_CalibratedGyroY_Dps : Outport  Port=3
  VVMC_CalibratedGyroZ_Dps : Outport  Port=4
  VVMC_CalibratedAccX_G : Outport  Port=5
  VVMC_CalibratedAccY_G : Outport  Port=6
  VVMC_CalibratedAccZ_G : Outport  Port=7
  wires:
  VINP_MemOffsetGyroX_raw16/1 -> [VINP_MemOffsetGyroX_raw16]
  VINP_MemOffsetGyroY_raw16/1 -> [VINP_MemOffsetGyroY_raw16]
  VINP_MemOffsetGyroZ_raw16/1 -> [VINP_MemOffsetGyroZ_raw16]
  VINP_MemOffsetAccX_raw16/1 -> [VINP_MemOffsetAccX_raw16]
  VINP_MemOffsetAccY_raw16/1 -> [VINP_MemOffsetAccY_raw16]
  VINP_MemOffsetAccZ_raw16/1 -> [VINP_MemOffsetAccZ_raw16]
  VINP_SensingGyroX_raw16/1 -> [VINP_SensingGyroX_raw16]
  VINP_SensingGyroY_raw16/1 -> [VINP_SensingGyroY_raw16]
  VINP_SensingGyroZ_raw16/1 -> [VINP_SensingGyroZ_raw16]
  VINP_SensingAccX_raw16/1 -> [VINP_SensingAccX_raw16]
  VINP_SensingAccY_raw16/1 -> [VINP_SensingAccY_raw16]
  VINP_SensingAccZ_raw16/1 -> [VINP_SensingAccZ_raw16]
  [VINP_MemOffsetGyroX_raw16] -> IMU memorized offset result/1(VINP_MemOffsetGyroX_raw16)
  [VINP_MemOffsetGyroY_raw16] -> IMU memorized offset result/2(VINP_MemOffsetGyroY_raw16)
  [VINP_MemOffsetGyroZ_raw16] -> IMU memorized offset result/3(VINP_MemOffsetGyroZ_raw16)
  [VINP_MemOffsetAccX_raw16] -> IMU memorized offset result/4(VINP_MemOffsetAccX_raw16)
  [VINP_MemOffsetAccY_raw16] -> IMU memorized offset result/5(VINP_MemOffsetAccY_raw16)
  [VINP_MemOffsetAccZ_raw16] -> IMU memorized offset result/6(VINP_MemOffsetAccZ_raw16)
  IMU memorized offset result/6(VVMC_MemOffsetAccZ_G) -> [VVMC_MemOffsetAccZ_G]
  IMU memorized offset result/5(VVMC_MemOffsetAccY_G) -> [VVMC_MemOffsetAccY_G]
  IMU memorized offset result/4(VVMC_MemOffsetAccX_G) -> [VVMC_MemOffsetAccX_G]
  IMU memorized offset result/3(VVMC_MemOffsetGyroZ_Dps) -> [VVMC_MemOffsetGyroZ_Dps]
  IMU memorized offset result/2(VVMC_MemOffsetGyroY_Dps) -> [VVMC_MemOffsetGyroY_Dps]
  IMU memorized offset result/1(VVMC_MemOffsetGyroX_Dps) -> [VVMC_MemOffsetGyroX_Dps]
  [VVMC_MemOffsetGyroY_Dps] -> "IMU sensing result "/8(VVMC_MemOffsetGyroY_Dps)
  [VVMC_MemOffsetAccX_G] -> "IMU sensing result "/10(VVMC_MemOffsetAccX_G)
  [VVMC_MemOffsetGyroZ_Dps] -> "IMU sensing result "/9(VVMC_MemOffsetGyroZ_Dps)
  [VVMC_MemOffsetAccY_G] -> "IMU sensing result "/11(VVMC_MemOffsetAccY_G)
  [VVMC_MemOffsetGyroX_Dps] -> "IMU sensing result "/7(VVMC_MemOffsetGyroX_Dps)
  [VVMC_MemOffsetAccZ_G] -> "IMU sensing result "/12(VVMC_MemOffsetAccZ_G)
  [VINP_SensingGyroX_raw16] -> "IMU sensing result "/1(VINP_SensingGyroX_raw16)
  [VINP_SensingAccZ_raw16] -> "IMU sensing result "/6(VINP_SensingAccZ_raw16)
  [VINP_SensingAccY_raw16] -> "IMU sensing result "/5(VINP_SensingAccY_raw16)
  [VINP_SensingAccX_raw16] -> "IMU sensing result "/4(VINP_SensingAccX_raw16)
  [VINP_SensingGyroZ_raw16] -> "IMU sensing result "/3(VINP_SensingGyroZ_raw16)
  [VINP_SensingGyroY_raw16] -> "IMU sensing result "/2(VINP_SensingGyroY_raw16)
  Constant/1 -> [VVMC_IMUEnaCmd_flg]  "VVMC_IMUEnaCmd_flg"
  [VVMC_IMUEnaCmd_flg] -> VVMC_IMUEnaCmd_flg/1
  task_time_s/1 -> [task_time_s]
  [task_time_s] -> "IMU sensing result "/13(task_time_s)
  "IMU sensing result "/1(VVMC_CalibratedGyroX_Dps) -> [VVMC_CalibratedGyroX_Dps]
  "IMU sensing result "/4(VVMC_CalibratedAccX_G) -> [VVMC_CalibratedAccX_G]
  "IMU sensing result "/5(VVMC_CalibratedAccY_G) -> [VVMC_CalibratedAccY_G]
  "IMU sensing result "/6(VVMC_CalibratedAccZ_G) -> [VVMC_CalibratedAccZ_G]
  "IMU sensing result "/2(VVMC_CalibratedGyroY_Dps) -> [VVMC_CalibratedGyroY_Dps]
  "IMU sensing result "/3(VVMC_CalibratedGyroZ_Dps) -> [VVMC_CalibratedGyroZ_Dps]
  [VVMC_CalibratedAccX_G] -> VVMC_CalibratedAccX_G/1
  [VVMC_CalibratedGyroX_Dps] -> VVMC_CalibratedGyroX_Dps/1
  [VVMC_CalibratedAccZ_G] -> VVMC_CalibratedAccZ_G/1
  [VVMC_CalibratedGyroZ_Dps] -> VVMC_CalibratedGyroZ_Dps/1
  [VVMC_CalibratedAccY_G] -> VVMC_CalibratedAccY_G/1
  [VVMC_CalibratedGyroY_Dps] -> VVMC_CalibratedGyroY_Dps/1

== system vmc/VMC/VMC/LFCAOIControl ==
  VINP_APSVRqEPASCtrl_flg : Inport
  VINP_APSRqEPASCtrl_flg : Inport  Port=2
  VINP_ADASStrWhlAngCtrlStatus_flg : Inport  Port=3
  VINP_APSAngleTarget_Deg : Inport  Port=4
  VINP_ADASDesStrWhlAngCtrlCmd_Deg : Inport  Port=5
  VINP_ADASAngCtrlTqWeightGain_pct : Inport  Port=6
  VINP_ADASDrvInputTqBoostAct_flg : Inport  Port=7
  VINP_ADASMaxAngCtrlOutTqLimit_Nm : Inport  Port=8
  VINP_ADASDrvInputTqBoostGain_pct : Inport  Port=9
  VINP_VehicleType_enum : Inport  Port=10
  VDDM_VMCLatCtrlProhibited_flg : Inport  Port=11
  VDDM_VMCEPSErr_flg : Inport  Port=12
  AND : Logic  AllPortsSameDT=off  OutDataTypeStr=boolean
  AND1 : Logic  AllPortsSameDT=off  OutDataTypeStr=boolean
  AND2 : Logic  AllPortsSameDT=off  OutDataTypeStr=boolean
  Cast To Boolean : DataTypeConversion  OutDataTypeStr=boolean
  Cast To Single : DataTypeConversion  OutDataTypeStr=single
  Cast To Single32 : DataTypeConversion  OutDataTypeStr=single
  Constant{1,4,10,12..13} (5 alike) : Constant  Value=ZERO_FLOAT
  Constant11 : Constant  Value=FALSE
  Constant2 : Constant  Value=KVMC_ADASAngCtrlTqWtGnUpperLim_pct
  Constant3 : Constant  Value=KVMC_ADASAngCtrlTqWtGnLowerLim_pct
  Constant5 : Constant  Value=TRUE
  Constant6 : Constant  Value=ENUM_VEHICLETYPE_D31HAWD
  Constant7 : Constant  Value=FALSE
  Constant8 : Constant  Value=ENUM_VEHICLETYPE_D31HRWD
  Constant9 : Constant  Value=FALSE
  Equal1 : RelationalOperator  Operator===  OutDataTypeStr=boolean  RndMeth=Simplest
  Equal3 : RelationalOperator  Operator===  OutDataTypeStr=boolean  RndMeth=Simplest
  NOT : Logic  Operator=NOT  AllPortsSameDT=off  OutDataTypeStr=boolean
  OR : Logic  Operator=OR  AllPortsSameDT=off  OutDataTypeStr=boolean
  OR1 : Logic  AllPortsSameDT=off  OutDataTypeStr=boolean
  OR2 : Logic  Operator=OR  AllPortsSameDT=off  OutDataTypeStr=boolean
  Saturation Dynamic3 : simulink/Discontinuities/Saturation Dynamic  OutMin=[]  OutMax=[]  OutDataTypeStr=Inherit: Same as second input  OutDataType=fixdt(1, 16)  OutScaling=2^-10  DoSatur=off
  Switch{1..6,9..13} (11 alike) : Switch  Criteria=u2 > Threshold
  VVMC_FDCVMCAPSVRqEPSCtrl_flg : Outport
  VVMC_FDCVMCAPSRqEPSCtrl_flg : Outport  Port=2
  VVMC_FDCVMCAPSAngleTarget_deg : Outport  Port=3
  VVMC_FDCVMCAngCtrlTqWtGn_pct : Outport  Port=4
  VVMC_FDCVMCDrInpTqBstAct_flg : Outport  Port=5
  VVMC_FDCVMCMaxAngCtrlOutTqLim_Nm : Outport  Port=6
  VVMC_FDCVMCDrInpTqBstGn_pct : Outport  Port=7
  wires:
  [VINP_APSAngleTarget_Deg] -> Switch9/1
  Switch11/1 -> Switch9/3
  AND/1 -> Switch11/2
  Switch12/1 -> [VVMC_FDCVMCAngCtrlTqWtGn_pct]  "VVMC_FDCVMCAngCtrlTqWtGn_pct"
  Switch9/1 -> [VVMC_FDCVMCAPSAngleTarget_deg]  "VVMC_FDCVMCAPSAngleTarget_deg"
  Cast To Single/1 -> [VVMC_FDCVMCMaxAngCtrlOutTqLim_Nm]  "VVMC_FDCVMCMaxAngCtrlOutTqLim_Nm"
  [VINP_APSRqEPASCtrl_flg] -> Switch10/2
  Switch2/1 -> Switch10/3
  Cast To Single32/1 -> [VVMC_FDCVMCDrInpTqBstGn_pct]  "VVMC_FDCVMCDrInpTqBstGn_pct"
  [VINP_APSRqEPASCtrl_flg] -> Switch12/2
  Switch10/1 -> [VVMC_FDCVMCAPSRqEPSCtrl_flg]  "VVMC_FDCVMCAPSRqEPSCtrl_flg"
  [VINP_ADASDesStrWhlAngCtrlCmd_Deg] -> Switch11/1
  Constant4/1 -> Switch11/3
  Equal3/1 -> OR/1
  [VINP_APSRqEPASCtrl_flg] -> Switch10/1
  [VINP_VehicleType_enum] -> Equal3/1
  Switch13/1 -> [VVMC_FDCVMCAPSVRqEPSCtrl_flg]  "VVMC_FDCVMCAPSVRqEPSCtrl_flg"
  Constant1/1 -> Switch12/1
  Constant2/1 -> Saturation Dynamic3/1
  [VINP_APSVRqEPASCtrl_flg] -> Switch4/3, OR2/1
  [VINP_ADASAngCtrlTqWeightGain_pct] -> Saturation Dynamic3/2
  Constant3/1 -> Saturation Dynamic3/3
  Cast To Boolean/1 -> [VVMC_FDCVMCDrInpTqBstAct_flg]  "VVMC_FDCVMCDrInpTqBstAct_flg"
  [VINP_APSRqEPASCtrl_flg] -> Switch9/2
  Switch3/1 -> Switch12/3
  [VINP_ADASDrvInputTqBoostAct_flg] -> AND1/1
  Constant8/1 -> Equal3/2
  Constant5/1 -> Switch1/1
  VINP_APSRqEPASCtrl_flg/1 -> [VINP_APSRqEPASCtrl_flg]
  VINP_APSVRqEPASCtrl_flg/1 -> [VINP_APSVRqEPASCtrl_flg]
  VINP_ADASMaxAngCtrlOutTqLimit_Nm/1 -> [VINP_ADASMaxAngCtrlOutTqLimit_Nm]
  VINP_ADASDrvInputTqBoostAct_flg/1 -> [VINP_ADASDrvInputTqBoostAct_flg]
  VINP_ADASAngCtrlTqWeightGain_pct/1 -> [VINP_ADASAngCtrlTqWeightGain_pct]
  VINP_ADASDesStrWhlAngCtrlCmd_Deg/1 -> [VINP_ADASDesStrWhlAngCtrlCmd_Deg]
  VINP_APSAngleTarget_Deg/1 -> [VINP_APSAngleTarget_Deg]
  VINP_ADASStrWhlAngCtrlStatus_flg/1 -> [VINP_ADASStrWhlAngCtrlStatus_flg]
  VINP_ADASDrvInputTqBoostGain_pct/1 -> [VINP_ADASDrvInputTqBoostGain_pct]
  VINP_VehicleType_enum/1 -> [VINP_VehicleType_enum]
  [VVMC_FDCVMCAPSVRqEPSCtrl_flg] -> VVMC_FDCVMCAPSVRqEPSCtrl_flg/1
  [VVMC_FDCVMCAPSRqEPSCtrl_flg] -> VVMC_FDCVMCAPSRqEPSCtrl_flg/1
  [VVMC_FDCVMCAPSAngleTarget_deg] -> VVMC_FDCVMCAPSAngleTarget_deg/1
  [VVMC_FDCVMCDrInpTqBstGn_pct] -> VVMC_FDCVMCDrInpTqBstGn_pct/1
  [VVMC_FDCVMCMaxAngCtrlOutTqLim_Nm] -> VVMC_FDCVMCMaxAngCtrlOutTqLim_Nm/1
  [VVMC_FDCVMCDrInpTqBstAct_flg] -> VVMC_FDCVMCDrInpTqBstAct_flg/1
  [VVMC_FDCVMCAngCtrlTqWtGn_pct] -> VVMC_FDCVMCAngCtrlTqWtGn_pct/1
  Constant6/1 -> Equal1/2
  [VINP_VehicleType_enum] -> Equal1/1
  Equal1/1 -> OR/2
  OR1/1 -> [VVMC_LFCAOIVehType_flg]  "VVMC_LFCAOIVehType_flg"
  [VVMC_LFCAOIVehType_flg] -> Switch1/2
  Switch1/1 -> Switch13/3
  Constant7/1 -> Switch1/3
  Constant9/1 -> Switch2/3
  [VVMC_LFCAOIVehType_flg] -> Switch2/2
  [VINP_ADASStrWhlAngCtrlStatus_flg] -> Switch2/1
  [VINP_ADASStrWhlAngCtrlStatus_flg] -> AND/1
  [VVMC_LFCAOIVehType_flg] -> AND/2
  [VVMC_LFCAOIVehType_flg] -> AND2/2
  [VINP_ADASStrWhlAngCtrlStatus_flg] -> AND2/1
  Constant10/1 -> Switch3/3
  AND2/1 -> Switch3/2
  Saturation Dynamic3/1 -> Switch3/1
  AND1/1 -> Cast To Boolean/1
  [VVMC_LFCAOIVehType_flg] -> AND1/2
  Switch5/1 -> Cast To Single/1
  Switch6/1 -> Cast To Single32/1
  VDDM_VMCLatCtrlProhibited_flg/1 -> [VDDM_VMCLatCtrlProhibited_flg]
  [VDDM_VMCLatCtrlProhibited_flg] -> NOT/1
  OR/1 -> OR1/1
  NOT/1 -> OR1/2
  VDDM_VMCEPSErr_flg/1 -> [VDDM_VMCEPSErr_flg]
  [VDDM_VMCEPSErr_flg] -> OR2/2
  OR2/1 -> Switch13/2
  Switch4/1 -> Switch13/1
  [VDDM_VMCEPSErr_flg] -> Switch4/2
  Constant11/1 -> Switch4/1
  Constant12/1 -> Switch5/3
  [VINP_ADASMaxAngCtrlOutTqLimit_Nm] -> Switch5/1
  Constant13/1 -> Switch6/3
  [VINP_ADASDrvInputTqBoostGain_pct] -> Switch6/1
  [VVMC_LFCAOIVehType_flg] -> Switch6/2
  [VVMC_LFCAOIVehType_flg] -> Switch5/2

== system vmc/VMC/VMC/Long Acceleration Calculation ==
  VINP_GRADE_Deg : Inport
  VINP_LongAccel_Gps : Inport  Port=2
  VINP_VehSpeed_kph : Inport  Port=3
  task_time_s : Inport  Port=4
  VVMC_EstSlopeCal_Deg : Inport  Port=5
  VVMC_FeatSetSpdForCalcu_kph : Inport  Port=6
  VVMC_LongAccelCalcuByVehSpdRaw_gps : Inport  Port=7
  VINP_DIDGetDynoMode_flg : Inport  Port=8
  AND2 : Logic  AllPortsSameDT=off  OutDataTypeStr=boolean
  AND5 : Logic  AllPortsSameDT=off  OutDataTypeStr=boolean
  Abs : Abs
  Add2 : Sum  Inputs=+-
  Add9 : Sum
  Cast To Single : DataTypeConversion  OutDataTypeStr=single
  Cast To Single1 : DataTypeConversion  OutDataTypeStr=single
  Cast To Single2 : DataTypeConversion  OutDataTypeStr=single
  Constant : Constant  Value=KVMC_GradeSourceSW_flg
  Constant{1,17,22,24} (4 alike) : Constant  Value=ZERO_FLOAT
  Constant14 : Constant  Value=KVMC_LongAccSource_enum
  Constant15 : Constant  Value=4  OutDataTypeStr=uint8
  Constant19 : Constant  Value=KVMC_DIDGetDynoModeSW_flg
  Constant2 : Constant  Value=KVMC_Veh2MetSpdLowBand_kph
  Constant23 : Constant  Value=KVMC_GradeInvalidValue_deg
  Constant27 : Constant  Value=KVMC_AccBWFilterCutOffFreq_raw32
  Constant29 : Constant  Value=C_TASK_10MS_S
  Constant3 : Constant  Value=KVMC_Veh2MetSpdHiBand_kph
  Data Type Conversion : DataTypeConversion  OutDataTypeStr=single
  Degrees to Radians1 : simulink_extras/Transformations/Degrees to Radians
  Equal4 : RelationalOperator  Operator===  OutDataTypeStr=boolean  RndMeth=Simplest
  FirstOrderFilter : hcu_lib/Basic_Blocks/FirstOrderFilter
  FirstOrderFilter8 : hcu_lib/Basic_Blocks/FirstOrderFilter
  MVMC_ACCLongSteadyCtrl_Y_kph : Lookup_n-D  NumberOfTableDimensions=1  BreakpointsForDimension1=AVMC_ACCLongSteadyCtrl_X_kph  Table=MVMC_ACCLongSteadyCtrl_Y_kph  ExtrapMethod=Clip  InternalRulePriority=Speed  RndMeth=Simplest  InputSameDT=on
  MVMC_CCLongSteadyCtrl_Y_kph : Lookup_n-D  NumberOfTableDimensions=1  BreakpointsForDimension1=AVMC_CCLongSteadyCtrl_X_kph  Table=MVMC_CCLongSteadyCtrl_Y_kph  ExtrapMethod=Clip  InternalRulePriority=Speed  RndMeth=Simplest  InputSameDT=on
  MVMC_LongAccDeadZone_Y_Gps : Lookup_n-D  NumberOfTableDimensions=1  BreakpointsForDimension1=AVMC_LongAccDeadZone_X_kph  Table=MVMC_LongAccDeadZone_Y_Gps  InternalRulePriority=Speed  RndMeth=Simplest  InputSameDT=on
  MVMC_LongAccFiltTsforP2_Y_c : Lookup_n-D  NumberOfTableDimensions=1  BreakpointsForDimension1=AVMC_LongAccFiltTsforP2_X_Gps  Table=MVMC_LongAccFiltTsforP2_Y_c  InternalRulePriority=Speed  RndMeth=Simplest  InputSameDT=on
  MVMC_MSALongSteadyCtrl_Y_kph : Lookup_n-D  NumberOfTableDimensions=1  BreakpointsForDimension1=AVMC_MSALongSteadyCtrl_X_kph  Table=MVMC_MSALongSteadyCtrl_Y_kph  ExtrapMethod=Clip  InternalRulePriority=Speed  RndMeth=Simplest  InputSameDT=on
  Relational Operator : RelationalOperator  Operator=>  OutDataTypeStr=boolean  RndMeth=Simplest
  Relational Operator2 : RelationalOperator  Operator=<=  OutDataTypeStr=boolean  RndMeth=Simplest
  Relational Operator5 : RelationalOperator  OutDataTypeStr=boolean  RndMeth=Simplest
  Relational Operator6 : RelationalOperator  Operator=<=  OutDataTypeStr=boolean  RndMeth=Simplest
  Sin1 : Trigonometry
  Switch{,1,7..8,14,16..17} (7 alike) : Switch  Criteria=u2 > Threshold
  Switch11 : Switch  Criteria=u2 > Threshold  Threshold=KVMC_LongAccelSWSpd_kph
  Switch15 : Switch  Criteria=u2 > Threshold  Threshold=KVMC_LongAccelSWSpd_kph
  Terminator : Terminator
  Vehicle to Meter Speed : Subsystem
  VVMC_LongAcc_Gps : Outport
  VVMC_EstSlope_Deg : Outport  Port=2
  wires:
  Cast To Single2/1 -> Switch1/3, Abs/1
  Constant1/1 -> Switch1/1
  [VVMC_LongAccDeadZone_Gps] -> Relational Operator2/2
  Abs/1 -> Relational Operator2/1
  Relational Operator2/1 -> Switch1/2
  [VINP_VehSpeed_kph] -> MVMC_LongAccDeadZone_Y_Gps/1
  MVMC_LongAccDeadZone_Y_Gps/1 -> [VVMC_LongAccDeadZone_Gps]  "VVMC_LongAccDeadZone_Gps"
  VINP_VehSpeed_kph/1 -> [VINP_VehSpeed_kph]
  Degrees to Radians1/1 -> Cast To Single/1
  Cast To Single1/1 -> Add2/1
  [VINP_GRADE_Deg] -> Switch/1
  Cast To Single/1 -> Sin1/1  "VVMC_GRADE_rad"
  Sin1/1 -> Add2/2  "VVMC_SINEGRADE_Gps"
  Add2/1 -> [VVMC_LongAccCal1_Gps]  "VVMC_LongAccCal1_Gps"
  [VINP_LongAccel_Gps] -> Cast To Single1/1
  VINP_GRADE_Deg/1 -> [VINP_GRADE_Deg]
  VINP_LongAccel_Gps/1 -> [VINP_LongAccel_Gps]
  [VVMC_LongAcc_Gps] -> VVMC_LongAcc_Gps/1
  [VINP_LongAccel_Gps] -> Switch8/3
  FirstOrderFilter/1 -> [VVMC_LongAcc_Gps]  "VVMC_LongAcc_Gps"
  MVMC_LongAccFiltTsforP2_Y_c/1 -> [VVMC_LongAccFiltTsforP2_c]  "VVMC_LongAccFiltTsforP2_c"
  [VINP_LongAccel_Gps] -> MVMC_LongAccFiltTsforP2_Y_c/1
  task_time_s/1 -> [task_time_s]
  Switch/1 -> Degrees to Radians1/1
  Constant/1 -> Switch/2
  [VVMC_EstSlope_Deg] -> Switch/3
  VVMC_EstSlopeCal_Deg/1 -> [VVMC_EstSlopeCal_Deg]
  Constant3/1 -> Relational Operator6/2
  Relational Operator6/1 -> AND2/2
  [VINP_VehSpeed_kph] -> Switch7/3
  Vehicle to Meter Speed/1(OutputSpeed) -> Switch7/1
  Relational Operator5/1 -> AND2/1
  [VINP_VehSpeed_kph] -> Relational Operator6/1
  [VINP_VehSpeed_kph] -> Vehicle to Meter Speed/1(InputSpeed)
  AND2/1 -> Switch7/2
  Switch7/1 -> [VVMC_CalMeterSpeed_kph]  "VVMC_CalMeterSpeed_kph"
  Constant2/1 -> Relational Operator5/2
  [VINP_VehSpeed_kph] -> Relational Operator5/1
  [VVMC_FeatSetSpdForCalcu_kph] -> MVMC_MSALongSteadyCtrl_Y_kph/1
  Data Type Conversion/1 -> MVMC_ACCLongSteadyCtrl_Y_kph/1
  MVMC_CCLongSteadyCtrl_Y_kph/1 -> [VVMC_CCLongSteadyCtrl_kph]  "VVMC_CCLongSteadyCtrl_kph"
  MVMC_MSALongSteadyCtrl_Y_kph/1 -> [VVMC_MSALongSteadyCtrl_kph]  "VVMC_MSALongSteadyCtrl_kph"
  MVMC_ACCLongSteadyCtrl_Y_kph/1 -> [VVMC_ACCLongSteadyCtrl_kph]  "VVMC_ACCLongSteadyCtrl_kph"
  [VVMC_FeatSetSpdForCalcu_kph] -> Data Type Conversion/1
  [VVMC_FeatSetSpdForCalcu_kph] -> MVMC_CCLongSteadyCtrl_Y_kph/1
  [VVMC_LongAccFiltTsforP2_c] -> FirstOrderFilter/3
  [task_time_s] -> FirstOrderFilter/2
  Switch1/1 -> FirstOrderFilter/1
  [VVMC_CalMeterSpeed_kph] -> Terminator/1
  VVMC_FeatSetSpdForCalcu_kph/1 -> [VVMC_FeatSetSpdForCalcu_kph]
  VVMC_LongAccelCalcuByVehSpdRaw_gps/1 -> [VVMC_LongAccelCalcuByVehSpdRaw_gps]
  Equal4/1 -> Switch8/2
  Constant15/1 -> Equal4/2
  Constant14/1 -> Equal4/1
  Switch8/1 -> Cast To Single2/1
  Constant29/1 -> Add9/1, FirstOrderFilter8/2
  [VINP_VehSpeed_kph] -> Switch11/2
  Add9/1 -> FirstOrderFilter8/3
  [VVMC_LongAccelCalcuByVehSpdRaw_gps] -> Switch11/1
  Switch11/1 -> FirstOrderFilter8/1
  Constant27/1 -> Add9/2
  FirstOrderFilter8/1 -> Switch8/1  "VVMC_LongAccelCalcuByVehSpd_gps"
  Constant17/1 -> Switch14/3
  [VVMC_LongAccCal1_Gps] -> Switch14/1
  [VINP_VehSpeed_kph] -> Switch14/2
  Switch14/1 -> Switch11/3
  [VVMC_EstSlope_Deg] -> VVMC_EstSlope_Deg/1
  VINP_DIDGetDynoMode_flg/1 -> [VINP_DIDGetDynoMode_flg]
  Relational Operator/1 -> Switch17/2
  [VVMC_EstSlopeCal_Deg] -> Switch15/1
  Constant23/1 -> Relational Operator/2
  [VINP_GRADE_Deg] -> Switch15/3
  Switch16/1 -> Relational Operator/1, Switch17/3
  [VINP_VehSpeed_kph] -> Switch15/2
  Switch15/1 -> Switch16/3
  Constant24/1 -> Switch17/1
  AND5/1 -> Switch16/2
  Constant22/1 -> Switch16/1
  Switch17/1 -> [VVMC_EstSlope_Deg]  "VVMC_EstSlope_Deg"
  Constant19/1 -> AND5/2
  [VINP_DIDGetDynoMode_flg] -> AND5/1
